simulink model "Lab10"  (R2016b)
settings: Solver=ode3  StartTime=0.0  StopTime=1.5  FixedStep=0.0001  RelTol=1e-3  EnableMultiTasking=on
settings Model: Creator=Niirn  LastModifiedBy=Niirn
settings DataIOCC: LimitDataPoints=on  SaveFormat=Array
settings OptimizationCC: LifeSpan=inf
settings DebuggingCC: UnderspecifiedInitializationDetection=Classic  MergeDetectMultiDrivingBlocksExec=none  SolverPrmCheckMsg=warning  SFUnexpectedBacktrackingDiag=warning  SFNoUnconditionalDefaultTransitionDiag=warning  SFExecutionAtInitializationDiag=none
settings HardwareCC: ProdBitPerPointer=32  ProdBitPerSizeT=32  ProdBitPerPtrDiffT=32  ProdLargestAtomicFloat=None  ProdIntDivRoundTo=Undefined  ProdEndianess=Unspecified  ProdWordSize=32  ProdHWDeviceType=32-bit Generic
settings ModelReferenceCC: PropagateSignalLabelsOutOfModel=off
settings GRTTargetCC: TargetLangStandard=C89/C90 (ANSI)  GeneratePreprocessorConditionals=Disable all
settings ConfigComp: CovMetricSettings=dw  CovHtmlReporting=on  CovSaveCumulativeToWorkspaceVar=on  CovSaveSingleToWorkspaceVar=on  CovExternalEMLEnable=off

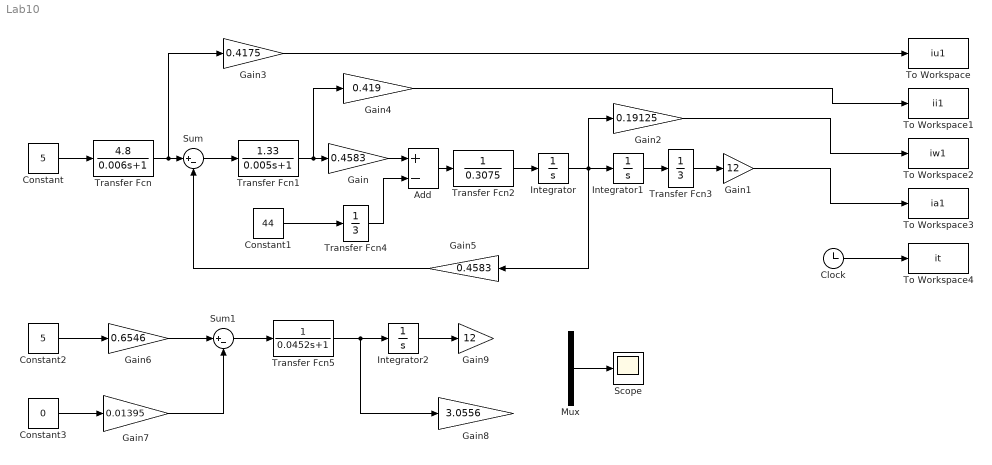
== system Lab10 ==
  Add : Sum  Inputs=+-
  Clock : Clock
  Constant : Constant  Value=5
  Constant1 : Constant  Value=44
  Constant2 : Constant  Value=5
  Constant3 : Constant  Value=0
  Gain : Gain  Gain=0.4583
  Gain1 : Gain  Gain=12
  Gain2 : Gain  Gain=0.19125
  Gain3 : Gain  Gain=0.4175
  Gain4 : Gain  Gain=0.419
  Gain5 : Gain  Gain=0.4583
  Gain6 : Gain  Gain=0.6546
  Gain7 : Gain  Gain=0.01395
  Gain8 : Gain  Gain=3.0556
  Gain9 : Gain  Gain=12
  Integrator : Integrator
  Integrator1 : Integrator
  Integrator2 : Integrator
  Mux : Mux
  Scope : Scope
  Sum : Sum  Inputs=|+-
  Sum1 : Sum  Inputs=|+-
  To Workspace : ToWorkspace  VariableName=iu1  SampleTime=-1
  To Workspace1 : ToWorkspace  VariableName=ii1  SampleTime=-1
  To Workspace2 : ToWorkspace  VariableName=iw1  SampleTime=-1
  To Workspace3 : ToWorkspace  VariableName=ia1  SampleTime=-1
  To Workspace4 : ToWorkspace  VariableName=it  SampleTime=-1
  Transfer Fcn : TransferFcn  Numerator=[4.8]  Denominator=[0.006 1]
  Transfer Fcn1 : TransferFcn  Numerator=[1.33]  Denominator=[0.005 1]
  Transfer Fcn2 : TransferFcn  Denominator=[0.3075]
  Transfer Fcn3 : TransferFcn  Denominator=[3]
  Transfer Fcn4 : TransferFcn  Denominator=[3]
  Transfer Fcn5 : TransferFcn  Denominator=[0.0452 1]
  wires:
  Constant1/1 -> Transfer Fcn4/1
  Constant/1 -> Transfer Fcn/1
  Transfer Fcn/1 -> Gain3/1, Sum/1
  Sum/1 -> Transfer Fcn1/1
  Transfer Fcn1/1 -> Gain4/1, Gain/1
  Gain/1 -> Add/1
  Transfer Fcn4/1 -> Add/2
  Add/1 -> Transfer Fcn2/1
  Transfer Fcn2/1 -> Integrator/1
  Integrator/1 -> Integrator1/1, Gain2/1, Gain5/1
  Integrator1/1 -> Transfer Fcn3/1
  Transfer Fcn3/1 -> Gain1/1
  Gain5/1 -> Sum/2
  Gain2/1 -> To Workspace2/1
  Gain4/1 -> To Workspace1/1
  Gain3/1 -> To Workspace/1
  Gain7/1 -> Sum1/2
  Gain6/1 -> Sum1/1
  Constant2/1 -> Gain6/1
  Constant3/1 -> Gain7/1
  Sum1/1 -> Transfer Fcn5/1
  Transfer Fcn5/1 -> Gain8/1, Integrator2/1
  Integrator2/1 -> Gain9/1
  Gain1/1 -> To Workspace3/1
  Mux/1 -> Scope/1
  Clock/1 -> To Workspace4/1
